simulink model "Verifica_LQR_DE6000008"  (R2025b)
settings: Solver=VariableStepAuto  StartTime=0.0  StopTime=10.0  RelTol=1e-3
undefined symbols (not defined in the file): K_LQR_i, K_LQR_x, r, x0_sylv
settings Model: Creator=salvo  LastModifiedBy=salvo

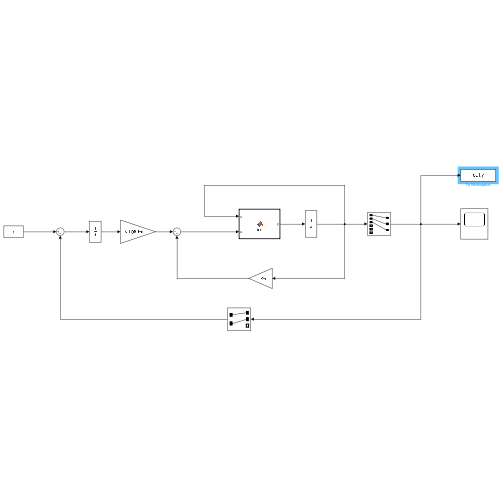
[thumbnail: Simulink's stored preview of the top-level diagram]
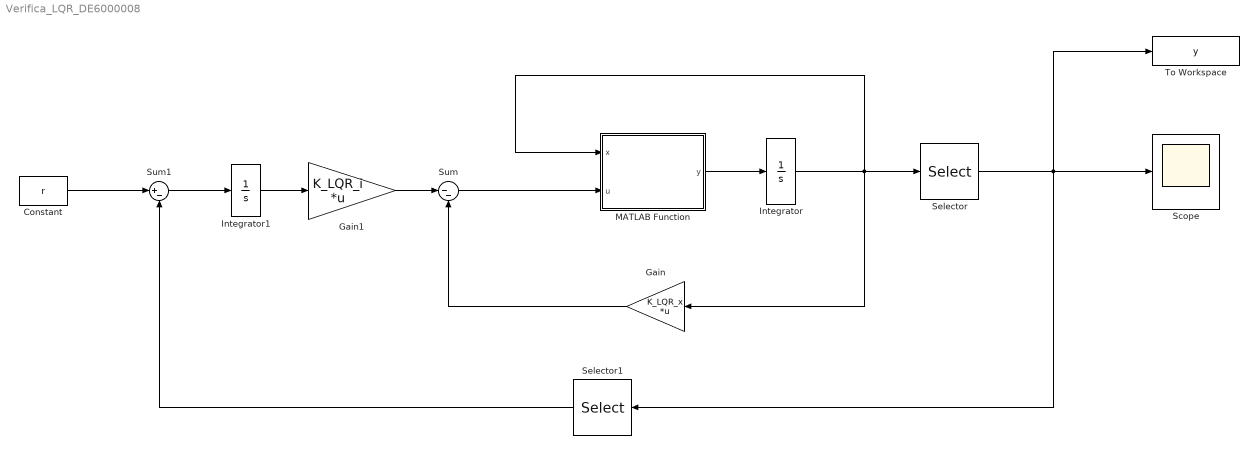
== system Verifica_LQR_DE6000008 ==
  Constant : Constant  Value=r
  Gain : Gain  Gain=K_LQR_x  Multiplication=Matrix(K*u)
  Gain1 : Gain  Gain=K_LQR_i  Multiplication=Matrix(K*u)
  Integrator : Integrator  InitialCondition=x0_sylv
  Integrator1 : Integrator
  MATLAB Function : MATLAB Function  TreatAsAtomicUnit=on
  Scope : Scope
      settings: ActiveDisplayYMinimum=-1.5134036451407038  ActiveDisplayYMaximum=11.2792670716823
  Selector : Selector  InputPortWidth=6  IndexOptions=Index vector (dialog)  Indices=[1 2 3]  OutputSizes=1
  Selector1 : Selector  InputPortWidth=3  IndexOptions=Index vector (dialog)  Indices=[1 2]  OutputSizes=1
  Sum : Sum  Inputs=|--
  Sum1 : Sum  Inputs=|+-
  To Workspace : ToWorkspace  VariableName=y  SaveFormat=Timeseries  SampleTime=-1
  wires:
  Integrator/1 -> Gain/1, Selector/1, MATLAB Function/1(x)
  MATLAB Function/1(y) -> Integrator/1
  Gain/1 -> Sum/2
  Sum/1 -> MATLAB Function/2(u)
  Gain1/1 -> Sum/1
  Selector/1 -> To Workspace/1, Selector1/1, Scope/1
  Integrator1/1 -> Gain1/1
  Sum1/1 -> Integrator1/1
  Constant/1 -> Sum1/1
  Selector1/1 -> Sum1/2

== matlab function Verifica_LQR_DE6000008/MATLAB Function ==
  data: x input; u input; y output
function y = fcn(x, u)

m = 1.5;
J = 0.025;
g = 9.81;

px = x(1);
pz = x(2);
theta = x(3);
dpx = x(4);
dpz = x(5);
dtheta = x(6);
    
T = u(1);
tau = u(2);
    
ddpx = -(T/m)*sin(theta);
ddpz = (T/m)*cos(theta) - g;
ddtheta = tau/J;
    
y = [dpx;
     dpz;
     dtheta;
     ddpx;
     ddpz;
     ddtheta];
